simulink model "Ultrafiltration"  (R2025b)
settings: Solver=FixedStepAuto  StartTime=0.0  StopTime=1440  FixedStep=1  RelTol=1e-3
InitFcn:
  | initUF
  | tic;
StartFcn:
  | disp("Start...")
StopFcn:
  | disp("Stop...")
  | fprintf("SimTime: %.02f min", toc/60)
values from neighbouring files (symbols this model uses):
  BW_Max_Time = 90    [initUF.m]
  BW_Max_Vol_gal = 5000    [initUF.m]
  CEB_Max_Time = 1000    [initUF.m]
  CEB_Max_Vol_gal = 5000    [initUF.m]
  CIP_Max_Time = 15000    [initUF.m]
undefined symbols (not defined in the file or in its folder): LUT
libraries: simulink x30
(part 2 of 5)

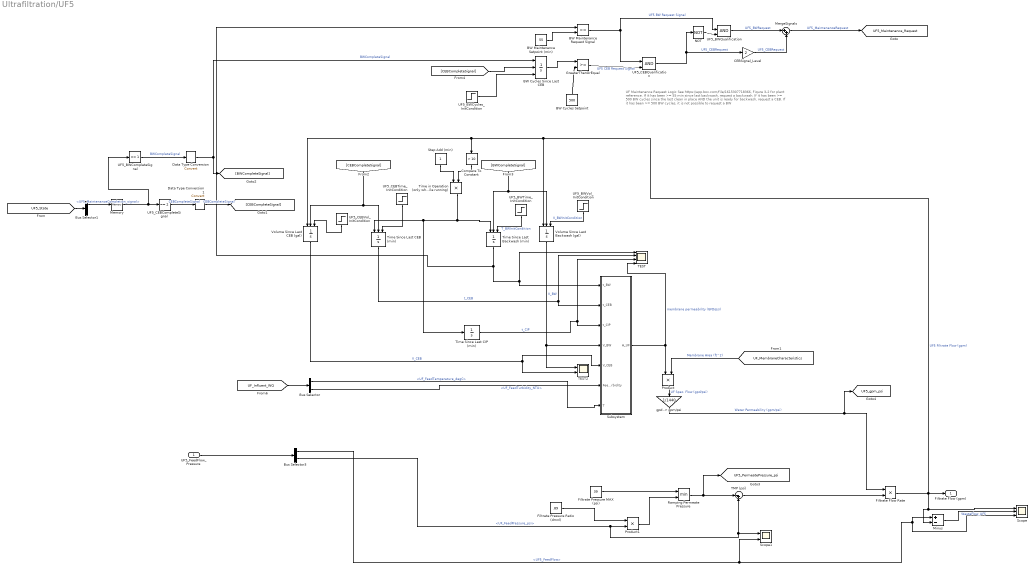
== system Ultrafiltration/UF5 ==
  note: UF Maintenance Request Logic
      | See https://app.box.com/file/1615307718366, Figure 3-2 for plant reference.
      |
      | If it has been >= 55 min since last backwash, request a backwash.
      | If it has been >= 500 BW cycles since the last clean in place AND the unit is ready for backwash, request a CEB.
      | If it has been >= 500 BW cycles, it is not possible to request a BW
  UF5_FeedFlow_Pressure : Inport
  BW Cycles Setpoint : Constant  Value=500
  BW Cycles Since Last CEB : Integrator  ExternalReset=rising  InitialConditionSource=external  InitialCondition=5
  BW Maintenance Request Signal : RelationalOperator  OutDataTypeStr=boolean  RndMeth=Simplest  InputSameDT=off
  BW Maintenance Setpoint (min) : Constant  Value=55
  Bus Selector : BusSelector  OutputSignals=UF_FeedTemperature_degC,UF_FeedTurbidity_NTU
  Bus Selector1 : BusSelector  OutputSignals=UF5_MaintenanceCompletion_signal,UF5_OperationsState_signal
  Bus Selector3 : BusSelector  OutputSignals=UF5_FeedFlow,UF_FeedPressure_psi
  CEBSignal_Level : Gain  Gain=2  OutDataTypeStr=double
  Compare To Constant : simulink/Logic and Bit Operations/Compare To Constant  relop=>  const=10  OutDataTypeStr=boolean
  Data Type Conversion : DataTypeConversion  SaturateOnIntegerOverflow=off  RndMeth=Floor
  Data Type Conversion1 : DataTypeConversion  SaturateOnIntegerOverflow=off  RndMeth=Floor
  Filtrate Flow Rate : Product
  Filtrate Pressure MAX (psi) : Constant  Value=39
  Filtrate Pressure Ratio (dmnl) : Constant  Value=.89
  GreaterThanOrEqual : RelationalOperator  OutDataTypeStr=boolean  RndMeth=Simplest  InputSameDT=off
  Memory : Memory
  MergeSignals : Sum  Inputs=|++
  Minus : Sum  Inputs=+-
  NOT : Logic  Operator=NOT  IconShape=distinctive  AllPortsSameDT=off  OutDataTypeStr=boolean
  Product : Product
  Product1 : Product
  Ramping Permeate Pressure : MinMax  Inputs=2
  Scope : Scope  NumInputPorts=3
      settings: ActiveDisplayYMinimum=-126.71796384165732  ActiveDisplayYMaximum=1140.4616745749161  DataLoggingVariableName=ScopeData10
  Scope1 : Scope  NumInputPorts=2
      settings: ActiveDisplayYMinimum=-129.2228584451866  ActiveDisplayYMaximum=1163.0057260066797  DataLoggingVariableName=ScopeData11
  Step Add (min) : Constant
  Subsystem : Subsystem
  TEST : Scope  NumInputPorts=4
      settings: ActiveDisplayYMinimum=13.625  ActiveDisplayYMaximum=27.375  DataLoggingVariableName=ScopeData3
  TEST2 : Scope  NumInputPorts=2
      settings: ActiveDisplayYMinimum=-311929.86683332996  ActiveDisplayYMaximum=2.8073688014999703E+6  DataLoggingVariableName=ScopeData4
  TMP (psi) : Sum  Inputs=|-+
  Time Since Last Backwash (min) : Integrator  ExternalReset=level hold  InitialConditionSource=external  InitialCondition=26
  Time Since Last CEB (min) : Integrator  ExternalReset=level hold  InitialConditionSource=external  InitialCondition=4833
  Time Since Last CIP (min) : Integrator  InitialCondition=round(CIP_Max_Time*rand())
  Time in Operation (only while running) : Product
  UF5_BWCompleteSignal : simulink/Logic and Bit Operations/Compare To Constant  relop===  const=1  OutDataTypeStr=uint8
  UF5_BWCycles_InitCondition : Step  Before=round(500 * rand())  After=0  SampleTime=0
  UF5_BWQualification : Logic  IconShape=distinctive  AllPortsSameDT=off  OutDataTypeStr=boolean
  UF5_BWTime_InitCondition : Step  Before=round(BW_Max_Time*rand())  After=0  SampleTime=0
  UF5_BWVol_InitCondition : Step  Before=round(BW_Max_Vol_gal*rand())  After=0  SampleTime=0
  UF5_CEBCompleteSignal : simulink/Logic and Bit Operations/Compare To Constant  relop===  const=2  OutDataTypeStr=uint8
  UF5_CEBQualification : Logic  IconShape=distinctive  AllPortsSameDT=off  OutDataTypeStr=boolean
  UF5_CEBTime_InitCondition : Step  Before=round(CEB_Max_Time*rand())  After=0  SampleTime=0
  UF5_CEBVol_InitCondition : Step  Before=round(CEB_Max_Vol_gal*rand())  After=0  SampleTime=0
  Volume Since Last Backwash (gal) : Integrator  ExternalReset=level hold  InitialConditionSource=external  InitialCondition=34330
  Volume Since Last CEB (gal) : Integrator  ExternalReset=rising  InitialConditionSource=external  InitialCondition=2777254
  "gpd -> gpm/psi" : Gain  Gain=1/1440
  Filtrate Flow (gpm) : Outport
  tag scope: UF5_Maintenance_Request=global, UF5_PermeatePressure_psi=global, UF5_gpm_psi=global
  wires:
  Volume Since Last Backwash (gal)/1 -> Subsystem/4(V_BW), TEST2/1  "V_BW"
  Time Since Last Backwash (min)/1 -> BW Maintenance Request Signal/1, Subsystem/1(t_BW), TEST/1
  Product/1 -> "gpd -> gpm/psi"/1  "UF Spec. Flow (gpd/psi)"
  [UF_MembraneCharacteristics] -> Product/2  "Membrane Area (ft^2)"
  "gpd -> gpm/psi"/1 -> Filtrate Flow Rate/1, [UF5_gpm_psi]  "Water Permeability (gpm/psi)"
  Time in Operation (only while running)/1 -> Time Since Last Backwash (min)/1, Time Since Last CEB (min)/1, Time Since Last CIP (min)/1
  Filtrate Flow Rate/1 -> Scope/1, Minus/2, Volume Since Last Backwash (gal)/1, Volume Since Last CEB (gal)/1, Compare To Constant/1, Filtrate Flow (gpm)/1  "UF5 Filtrate Flow (gpm)"
  Time Since Last CEB (min)/1 -> Subsystem/2(t_CEB), TEST/2  "t_CEB"
  Volume Since Last CEB (gal)/1 -> Subsystem/5(V_CEB), TEST2/2  "V_CEB"
  Time Since Last CIP (min)/1 -> Subsystem/3(t_CIP), TEST/3  "t_CIP"
  Filtrate Pressure MAX (psi)/1 -> Ramping Permeate Pressure/1
  [UF_Influent_WQ] -> Bus Selector/1
  Bus Selector/1 -> Subsystem/7(T)  "<UF_FeedTemperature_degC>"
  UF5_FeedFlow_Pressure/1 -> Bus Selector3/1
  Filtrate Pressure Ratio (dmnl)/1 -> Product1/1
  Product1/1 -> Ramping Permeate Pressure/2
  Ramping Permeate Pressure/1 -> [UF5_PermeatePressure_psi], TMP (psi)/1
  TMP (psi)/1 -> Filtrate Flow Rate/2
  BW Maintenance Setpoint (min)/1 -> BW Maintenance Request Signal/2
  BW Cycles Since Last CEB/1 -> GreaterThanOrEqual/1
  BW Cycles Setpoint/1 -> GreaterThanOrEqual/2
  Bus Selector/2 -> Subsystem/6(Feed Turbidity)  "<UF_FeedTurbidity_NTU>"
  [UF5_State] -> Bus Selector1/1
  MergeSignals/1 -> [UF5_Maintenance_Request]  "UF5_MaintenanceRequest"
  UF5_CEBCompleteSignal/1 -> Data Type Conversion1/1  "CEBCompleteSignal"
  [CEBCompleteSignal] -> Volume Since Last CEB (gal)/2, Time Since Last CEB (min)/2
  Data Type Conversion/1 -> [BWCompleteSignal], BW Cycles Since Last CEB/1  "BWCompleteSignal"
  [BWCompleteSignal] -> Volume Since Last Backwash (gal)/2, Time Since Last Backwash (min)/2
  [CEBCompleteSignal] -> BW Cycles Since Last CEB/2
  Bus Selector1/1 -> Memory/1  "<UF5_MaintenanceCompletion_signal>"
  UF5_BWCompleteSignal/1 -> Data Type Conversion/1  "BWCompleteSignal"
  Data Type Conversion1/1 -> [CEBCompleteSignal]  "CEBCompleteSignal"
  UF5_BWCycles_InitCondition/1 -> BW Cycles Since Last CEB/3
  Subsystem/1(A_UF) -> TEST/4, Product/1  "membrane permeability (GFD/psi)"
  UF5_BWTime_InitCondition/1 -> Time Since Last Backwash (min)/3  "T_BWInitCondition"
  UF5_CEBVol_InitCondition/1 -> Volume Since Last CEB (gal)/3
  UF5_CEBTime_InitCondition/1 -> Time Since Last CEB (min)/3
  UF5_BWVol_InitCondition/1 -> Volume Since Last Backwash (gal)/3  "V_BWInitCondition"
  Step Add (min)/1 -> Time in Operation (only while running)/1
  Compare To Constant/1 -> Time in Operation (only while running)/2
  Memory/1 -> UF5_BWCompleteSignal/1, UF5_CEBCompleteSignal/1
  UF5_BWQualification/1 -> MergeSignals/1  "UF5_BWRequest"
  GreaterThanOrEqual/1 -> UF5_CEBQualification/2  "UF5 CEB Request Signal"
  UF5_CEBQualification/1 -> CEBSignal_Level/1, NOT/1  "UF5_CEBRequest"
  BW Maintenance Request Signal/1 -> UF5_BWQualification/1, UF5_CEBQualification/1  "UF5 BW Request Signal"
  NOT/1 -> UF5_BWQualification/2
  CEBSignal_Level/1 -> MergeSignals/2  "UF5_CEBRequest"
  Bus Selector3/1 -> Scope1/2, Minus/1, Scope/3  "<UF5_FeedFlow>"
  Bus Selector3/2 -> TMP (psi)/2, Scope1/1, Product1/2  "<UF_FeedPressure_psi>"
  Minus/1 -> Scope/2  "WasteFlow_UF5"

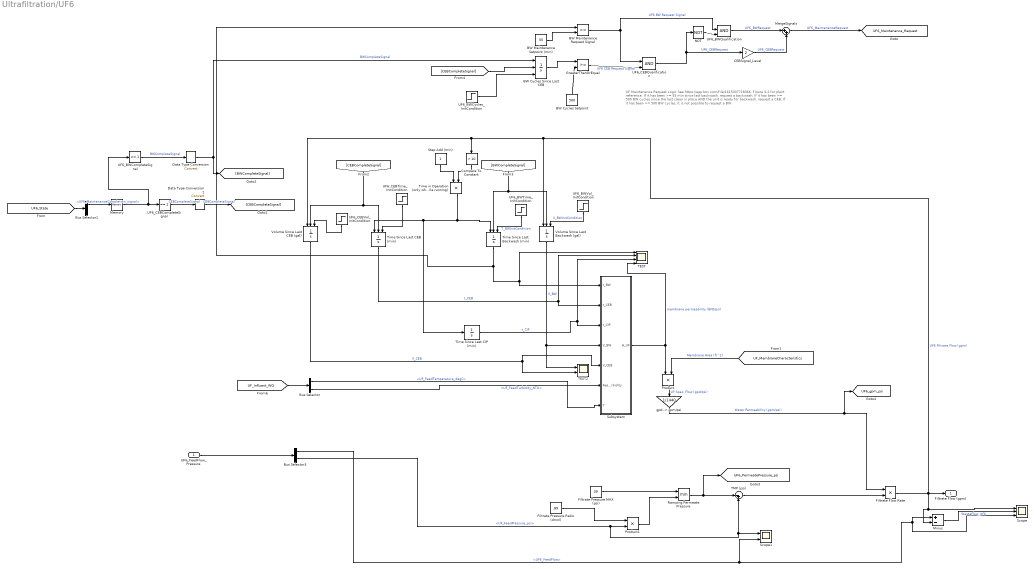
== system Ultrafiltration/UF6 ==
  note: UF Maintenance Request Logic
      | See https://app.box.com/file/1615307718366, Figure 3-2 for plant reference.
      |
      | If it has been >= 55 min since last backwash, request a backwash.
      | If it has been >= 500 BW cycles since the last clean in place AND the unit is ready for backwash, request a CEB.
      | If it has been >= 500 BW cycles, it is not possible to request a BW
  UF6_FeedFlow_Pressure : Inport
  BW Cycles Setpoint : Constant  Value=500
  BW Cycles Since Last CEB : Integrator  ExternalReset=rising  InitialConditionSource=external  InitialCondition=5
  BW Maintenance Request Signal : RelationalOperator  OutDataTypeStr=boolean  RndMeth=Simplest  InputSameDT=off
  BW Maintenance Setpoint (min) : Constant  Value=55
  Bus Selector : BusSelector  OutputSignals=UF_FeedTemperature_degC,UF_FeedTurbidity_NTU
  Bus Selector1 : BusSelector  OutputSignals=UF6_MaintenanceCompletion_signal,UF6_OperationsState_signal
  Bus Selector3 : BusSelector  OutputSignals=UF6_FeedFlow,UF_FeedPressure_psi
  CEBSignal_Level : Gain  Gain=2  OutDataTypeStr=double
  Compare To Constant : simulink/Logic and Bit Operations/Compare To Constant  relop=>  const=10  OutDataTypeStr=boolean
  Data Type Conversion : DataTypeConversion  SaturateOnIntegerOverflow=off  RndMeth=Floor
  Data Type Conversion1 : DataTypeConversion  SaturateOnIntegerOverflow=off  RndMeth=Floor
  Filtrate Flow Rate : Product
  Filtrate Pressure MAX (psi) : Constant  Value=39
  Filtrate Pressure Ratio (dmnl) : Constant  Value=.89
  GreaterThanOrEqual : RelationalOperator  OutDataTypeStr=boolean  RndMeth=Simplest  InputSameDT=off
  Memory : Memory
  MergeSignals : Sum  Inputs=|++
  Minus : Sum  Inputs=+-
  NOT : Logic  Operator=NOT  IconShape=distinctive  AllPortsSameDT=off  OutDataTypeStr=boolean
  Product : Product
  Product1 : Product
  Ramping Permeate Pressure : MinMax  Inputs=2
  Scope : Scope  NumInputPorts=3
      settings: ActiveDisplayYMinimum=-126.71796384165732  ActiveDisplayYMaximum=1140.4616745749161  DataLoggingVariableName=ScopeData10
  Scope1 : Scope  NumInputPorts=2
      settings: ActiveDisplayYMinimum=-129.2228584451866  ActiveDisplayYMaximum=1163.0057260066797  DataLoggingVariableName=ScopeData11
  Step Add (min) : Constant
  Subsystem : Subsystem
  TEST : Scope  NumInputPorts=4
      settings: ActiveDisplayYMinimum=13.625  ActiveDisplayYMaximum=27.375  DataLoggingVariableName=ScopeData3
  TEST2 : Scope  NumInputPorts=2
      settings: ActiveDisplayYMinimum=-311929.86683332996  ActiveDisplayYMaximum=2.8073688014999703E+6  DataLoggingVariableName=ScopeData4
  TMP (psi) : Sum  Inputs=|-+
  Time Since Last Backwash (min) : Integrator  ExternalReset=level hold  InitialConditionSource=external  InitialCondition=26
  Time Since Last CEB (min) : Integrator  ExternalReset=level hold  InitialConditionSource=external  InitialCondition=4833
  Time Since Last CIP (min) : Integrator  InitialCondition=round(CIP_Max_Time*rand())
  Time in Operation (only while running) : Product
  UF6_BWCompleteSignal : simulink/Logic and Bit Operations/Compare To Constant  relop===  const=1  OutDataTypeStr=uint8
  UF6_BWCycles_InitCondition : Step  Before=round(500 * rand())  After=0  SampleTime=0
  UF6_BWQualification : Logic  IconShape=distinctive  AllPortsSameDT=off  OutDataTypeStr=boolean
  UF6_BWTime_InitCondition : Step  Before=round(BW_Max_Time*rand())  After=0  SampleTime=0
  UF6_BWVol_InitCondition : Step  Before=round(BW_Max_Vol_gal*rand())  After=0  SampleTime=0
  UF6_CEBCompleteSignal : simulink/Logic and Bit Operations/Compare To Constant  relop===  const=2  OutDataTypeStr=uint8
  UF6_CEBQualification : Logic  IconShape=distinctive  AllPortsSameDT=off  OutDataTypeStr=boolean
  UF6_CEBTime_InitCondition : Step  Before=round(CEB_Max_Time*rand())  After=0  SampleTime=0
  UF6_CEBVol_InitCondition : Step  Before=round(CEB_Max_Vol_gal*rand())  After=0  SampleTime=0
  Volume Since Last Backwash (gal) : Integrator  ExternalReset=level hold  InitialConditionSource=external  InitialCondition=34330
  Volume Since Last CEB (gal) : Integrator  ExternalReset=rising  InitialConditionSource=external  InitialCondition=2777254
  "gpd -> gpm/psi" : Gain  Gain=1/1440
  Filtrate Flow (gpm) : Outport
  tag scope: UF6_Maintenance_Request=global, UF6_PermeatePressure_psi=global, UF6_gpm_psi=global
  wires:
  Volume Since Last Backwash (gal)/1 -> Subsystem/4(V_BW), TEST2/1  "V_BW"
  Time Since Last Backwash (min)/1 -> BW Maintenance Request Signal/1, Subsystem/1(t_BW), TEST/1
  Product/1 -> "gpd -> gpm/psi"/1  "UF Spec. Flow (gpd/psi)"
  [UF_MembraneCharacteristics] -> Product/2  "Membrane Area (ft^2)"
  "gpd -> gpm/psi"/1 -> Filtrate Flow Rate/1, [UF6_gpm_psi]  "Water Permeability (gpm/psi)"
  Time in Operation (only while running)/1 -> Time Since Last Backwash (min)/1, Time Since Last CEB (min)/1, Time Since Last CIP (min)/1
  Filtrate Flow Rate/1 -> Scope/1, Minus/2, Volume Since Last Backwash (gal)/1, Volume Since Last CEB (gal)/1, Compare To Constant/1, Filtrate Flow (gpm)/1  "UF6 Filtrate Flow (gpm)"
  Time Since Last CEB (min)/1 -> Subsystem/2(t_CEB), TEST/2  "t_CEB"
  Volume Since Last CEB (gal)/1 -> Subsystem/5(V_CEB), TEST2/2  "V_CEB"
  Time Since Last CIP (min)/1 -> Subsystem/3(t_CIP), TEST/3  "t_CIP"
  Filtrate Pressure MAX (psi)/1 -> Ramping Permeate Pressure/1
  [UF_Influent_WQ] -> Bus Selector/1
  Bus Selector/1 -> Subsystem/7(T)  "<UF_FeedTemperature_degC>"
  UF6_FeedFlow_Pressure/1 -> Bus Selector3/1
  Filtrate Pressure Ratio (dmnl)/1 -> Product1/1
  Product1/1 -> Ramping Permeate Pressure/2
  Ramping Permeate Pressure/1 -> [UF6_PermeatePressure_psi], TMP (psi)/1
  TMP (psi)/1 -> Filtrate Flow Rate/2
  BW Maintenance Setpoint (min)/1 -> BW Maintenance Request Signal/2
  BW Cycles Since Last CEB/1 -> GreaterThanOrEqual/1
  BW Cycles Setpoint/1 -> GreaterThanOrEqual/2
  Bus Selector/2 -> Subsystem/6(Feed Turbidity)  "<UF_FeedTurbidity_NTU>"
  [UF6_State] -> Bus Selector1/1
  MergeSignals/1 -> [UF6_Maintenance_Request]  "UF6_MaintenanceRequest"
  UF6_CEBCompleteSignal/1 -> Data Type Conversion1/1  "CEBCompleteSignal"
  [CEBCompleteSignal] -> Volume Since Last CEB (gal)/2, Time Since Last CEB (min)/2
  Data Type Conversion/1 -> [BWCompleteSignal], BW Cycles Since Last CEB/1  "BWCompleteSignal"
  [BWCompleteSignal] -> Volume Since Last Backwash (gal)/2, Time Since Last Backwash (min)/2
  [CEBCompleteSignal] -> BW Cycles Since Last CEB/2
  Bus Selector1/1 -> Memory/1  "<UF6_MaintenanceCompletion_signal>"
  UF6_BWCompleteSignal/1 -> Data Type Conversion/1  "BWCompleteSignal"
  Data Type Conversion1/1 -> [CEBCompleteSignal]  "CEBCompleteSignal"
  UF6_BWCycles_InitCondition/1 -> BW Cycles Since Last CEB/3
  Subsystem/1(A_UF) -> TEST/4, Product/1  "membrane permeability (GFD/psi)"
  UF6_BWTime_InitCondition/1 -> Time Since Last Backwash (min)/3  "T_BWInitCondition"
  UF6_CEBVol_InitCondition/1 -> Volume Since Last CEB (gal)/3
  UF6_CEBTime_InitCondition/1 -> Time Since Last CEB (min)/3
  UF6_BWVol_InitCondition/1 -> Volume Since Last Backwash (gal)/3  "V_BWInitCondition"
  Step Add (min)/1 -> Time in Operation (only while running)/1
  Compare To Constant/1 -> Time in Operation (only while running)/2
  Memory/1 -> UF6_BWCompleteSignal/1, UF6_CEBCompleteSignal/1
  UF6_BWQualification/1 -> MergeSignals/1  "UF6_BWRequest"
  GreaterThanOrEqual/1 -> UF6_CEBQualification/2  "UF6 CEB Request Signal"
  UF6_CEBQualification/1 -> CEBSignal_Level/1, NOT/1  "UF6_CEBRequest"
  BW Maintenance Request Signal/1 -> UF6_BWQualification/1, UF6_CEBQualification/1  "UF6 BW Request Signal"
  NOT/1 -> UF6_BWQualification/2
  CEBSignal_Level/1 -> MergeSignals/2  "UF6_CEBRequest"
  Bus Selector3/1 -> Scope1/2, Minus/1, Scope/3  "<UF6_FeedFlow>"
  Bus Selector3/2 -> TMP (psi)/2, Scope1/1, Product1/2  "<UF_FeedPressure_psi>"
  Minus/1 -> Scope/2  "WasteFlow_UF6"

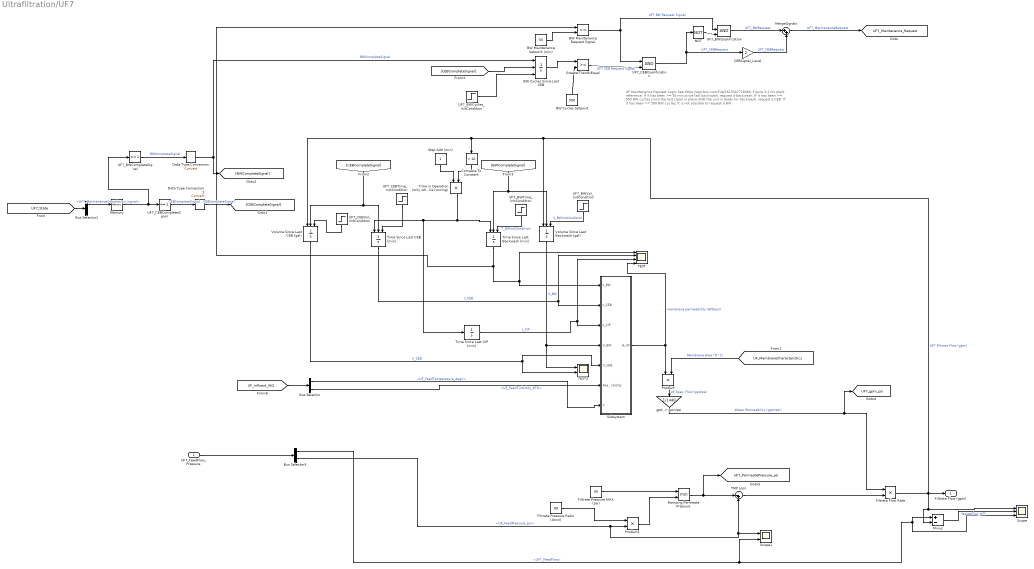
== system Ultrafiltration/UF7 ==
  note: UF Maintenance Request Logic
      | See https://app.box.com/file/1615307718366, Figure 3-2 for plant reference.
      |
      | If it has been >= 55 min since last backwash, request a backwash.
      | If it has been >= 500 BW cycles since the last clean in place AND the unit is ready for backwash, request a CEB.
      | If it has been >= 500 BW cycles, it is not possible to request a BW
  UF7_FeedFlow_Pressure : Inport
  BW Cycles Setpoint : Constant  Value=500
  BW Cycles Since Last CEB : Integrator  ExternalReset=rising  InitialConditionSource=external  InitialCondition=5
  BW Maintenance Request Signal : RelationalOperator  OutDataTypeStr=boolean  RndMeth=Simplest  InputSameDT=off
  BW Maintenance Setpoint (min) : Constant  Value=55
  Bus Selector : BusSelector  OutputSignals=UF_FeedTemperature_degC,UF_FeedTurbidity_NTU
  Bus Selector1 : BusSelector  OutputSignals=UF7_MaintenanceCompletion_signal,UF7_OperationsState_signal
  Bus Selector3 : BusSelector  OutputSignals=UF7_FeedFlow,UF_FeedPressure_psi
  CEBSignal_Level : Gain  Gain=2  OutDataTypeStr=double
  Compare To Constant : simulink/Logic and Bit Operations/Compare To Constant  relop=>  const=10  OutDataTypeStr=boolean
  Data Type Conversion : DataTypeConversion  SaturateOnIntegerOverflow=off  RndMeth=Floor
  Data Type Conversion1 : DataTypeConversion  SaturateOnIntegerOverflow=off  RndMeth=Floor
  Filtrate Flow Rate : Product
  Filtrate Pressure MAX (psi) : Constant  Value=39
  Filtrate Pressure Ratio (dmnl) : Constant  Value=.89
  GreaterThanOrEqual : RelationalOperator  OutDataTypeStr=boolean  RndMeth=Simplest  InputSameDT=off
  Memory : Memory
  MergeSignals : Sum  Inputs=|++
  Minus : Sum  Inputs=+-
  NOT : Logic  Operator=NOT  IconShape=distinctive  AllPortsSameDT=off  OutDataTypeStr=boolean
  Product : Product
  Product1 : Product
  Ramping Permeate Pressure : MinMax  Inputs=2
  Scope : Scope  NumInputPorts=3
      settings: ActiveDisplayYMinimum=-126.71796384165732  ActiveDisplayYMaximum=1140.4616745749161  DataLoggingVariableName=ScopeData10
  Scope1 : Scope  NumInputPorts=2
      settings: ActiveDisplayYMinimum=-129.2228584451866  ActiveDisplayYMaximum=1163.0057260066797  DataLoggingVariableName=ScopeData11
  Step Add (min) : Constant
  Subsystem : Subsystem
  TEST : Scope  NumInputPorts=4
      settings: ActiveDisplayYMinimum=13.625  ActiveDisplayYMaximum=27.375  DataLoggingVariableName=ScopeData3
  TEST2 : Scope  NumInputPorts=2
      settings: ActiveDisplayYMinimum=-311929.86683332996  ActiveDisplayYMaximum=2.8073688014999703E+6  DataLoggingVariableName=ScopeData4
  TMP (psi) : Sum  Inputs=|-+
  Time Since Last Backwash (min) : Integrator  ExternalReset=level hold  InitialConditionSource=external  InitialCondition=26
  Time Since Last CEB (min) : Integrator  ExternalReset=level hold  InitialConditionSource=external  InitialCondition=4833
  Time Since Last CIP (min) : Integrator  InitialCondition=round(CIP_Max_Time*rand())
  Time in Operation (only while running) : Product
  UF7_BWCompleteSignal : simulink/Logic and Bit Operations/Compare To Constant  relop===  const=1  OutDataTypeStr=uint8
  UF7_BWCycles_InitCondition : Step  Before=round(500 * rand())  After=0  SampleTime=0
  UF7_BWQualification : Logic  IconShape=distinctive  AllPortsSameDT=off  OutDataTypeStr=boolean
  UF7_BWTime_InitCondition : Step  Before=round(BW_Max_Time*rand())  After=0  SampleTime=0
  UF7_BWVol_InitCondition : Step  Before=round(BW_Max_Vol_gal*rand())  After=0  SampleTime=0
  UF7_CEBCompleteSignal : simulink/Logic and Bit Operations/Compare To Constant  relop===  const=2  OutDataTypeStr=uint8
  UF7_CEBQualification : Logic  IconShape=distinctive  AllPortsSameDT=off  OutDataTypeStr=boolean
  UF7_CEBTime_InitCondition : Step  Before=round(CEB_Max_Time*rand())  After=0  SampleTime=0
  UF7_CEBVol_InitCondition : Step  Before=round(CEB_Max_Vol_gal*rand())  After=0  SampleTime=0
  Volume Since Last Backwash (gal) : Integrator  ExternalReset=level hold  InitialConditionSource=external  InitialCondition=34330
  Volume Since Last CEB (gal) : Integrator  ExternalReset=rising  InitialConditionSource=external  InitialCondition=2777254
  "gpd -> gpm/psi" : Gain  Gain=1/1440
  Filtrate Flow (gpm) : Outport
  tag scope: UF7_Maintenance_Request=global, UF7_PermeatePressure_psi=global, UF7_gpm_psi=global
  wires:
  Volume Since Last Backwash (gal)/1 -> Subsystem/4(V_BW), TEST2/1  "V_BW"
  Time Since Last Backwash (min)/1 -> BW Maintenance Request Signal/1, Subsystem/1(t_BW), TEST/1
  Product/1 -> "gpd -> gpm/psi"/1  "UF Spec. Flow (gpd/psi)"
  [UF_MembraneCharacteristics] -> Product/2  "Membrane Area (ft^2)"
  "gpd -> gpm/psi"/1 -> Filtrate Flow Rate/1, [UF7_gpm_psi]  "Water Permeability (gpm/psi)"
  Time in Operation (only while running)/1 -> Time Since Last Backwash (min)/1, Time Since Last CEB (min)/1, Time Since Last CIP (min)/1
  Filtrate Flow Rate/1 -> Scope/1, Minus/2, Volume Since Last Backwash (gal)/1, Volume Since Last CEB (gal)/1, Compare To Constant/1, Filtrate Flow (gpm)/1  "UF7 Filtrate Flow (gpm)"
  Time Since Last CEB (min)/1 -> Subsystem/2(t_CEB), TEST/2  "t_CEB"
  Volume Since Last CEB (gal)/1 -> Subsystem/5(V_CEB), TEST2/2  "V_CEB"
  Time Since Last CIP (min)/1 -> Subsystem/3(t_CIP), TEST/3  "t_CIP"
  Filtrate Pressure MAX (psi)/1 -> Ramping Permeate Pressure/1
  [UF_Influent_WQ] -> Bus Selector/1
  Bus Selector/1 -> Subsystem/7(T)  "<UF_FeedTemperature_degC>"
  UF7_FeedFlow_Pressure/1 -> Bus Selector3/1
  Filtrate Pressure Ratio (dmnl)/1 -> Product1/1
  Product1/1 -> Ramping Permeate Pressure/2
  Ramping Permeate Pressure/1 -> [UF7_PermeatePressure_psi], TMP (psi)/1
  TMP (psi)/1 -> Filtrate Flow Rate/2
  BW Maintenance Setpoint (min)/1 -> BW Maintenance Request Signal/2
  BW Cycles Since Last CEB/1 -> GreaterThanOrEqual/1
  BW Cycles Setpoint/1 -> GreaterThanOrEqual/2
  Bus Selector/2 -> Subsystem/6(Feed Turbidity)  "<UF_FeedTurbidity_NTU>"
  [UF7_State] -> Bus Selector1/1
  MergeSignals/1 -> [UF7_Maintenance_Request]  "UF7_MaintenanceRequest"
  UF7_CEBCompleteSignal/1 -> Data Type Conversion1/1  "CEBCompleteSignal"
  [CEBCompleteSignal] -> Volume Since Last CEB (gal)/2, Time Since Last CEB (min)/2
  Data Type Conversion/1 -> [BWCompleteSignal], BW Cycles Since Last CEB/1  "BWCompleteSignal"
  [BWCompleteSignal] -> Volume Since Last Backwash (gal)/2, Time Since Last Backwash (min)/2
  [CEBCompleteSignal] -> BW Cycles Since Last CEB/2
  Bus Selector1/1 -> Memory/1  "<UF7_MaintenanceCompletion_signal>"
  UF7_BWCompleteSignal/1 -> Data Type Conversion/1  "BWCompleteSignal"
  Data Type Conversion1/1 -> [CEBCompleteSignal]  "CEBCompleteSignal"
  UF7_BWCycles_InitCondition/1 -> BW Cycles Since Last CEB/3
  Subsystem/1(A_UF) -> TEST/4, Product/1  "membrane permeability (GFD/psi)"
  UF7_BWTime_InitCondition/1 -> Time Since Last Backwash (min)/3  "T_BWInitCondition"
  UF7_CEBVol_InitCondition/1 -> Volume Since Last CEB (gal)/3
  UF7_CEBTime_InitCondition/1 -> Time Since Last CEB (min)/3
  UF7_BWVol_InitCondition/1 -> Volume Since Last Backwash (gal)/3  "V_BWInitCondition"
  Step Add (min)/1 -> Time in Operation (only while running)/1
  Compare To Constant/1 -> Time in Operation (only while running)/2
  Memory/1 -> UF7_BWCompleteSignal/1, UF7_CEBCompleteSignal/1
  UF7_BWQualification/1 -> MergeSignals/1  "UF7_BWRequest"
  GreaterThanOrEqual/1 -> UF7_CEBQualification/2  "UF7 CEB Request Signal"
  UF7_CEBQualification/1 -> CEBSignal_Level/1, NOT/1  "UF7_CEBRequest"
  BW Maintenance Request Signal/1 -> UF7_BWQualification/1, UF7_CEBQualification/1  "UF7 BW Request Signal"
  NOT/1 -> UF7_BWQualification/2
  CEBSignal_Level/1 -> MergeSignals/2  "UF7_CEBRequest"
  Bus Selector3/1 -> Scope1/2, Minus/1, Scope/3  "<UF7_FeedFlow>"
  Bus Selector3/2 -> TMP (psi)/2, Scope1/1, Product1/2  "<UF_FeedPressure_psi>"
  Minus/1 -> Scope/2  "WasteFlow_UF7"

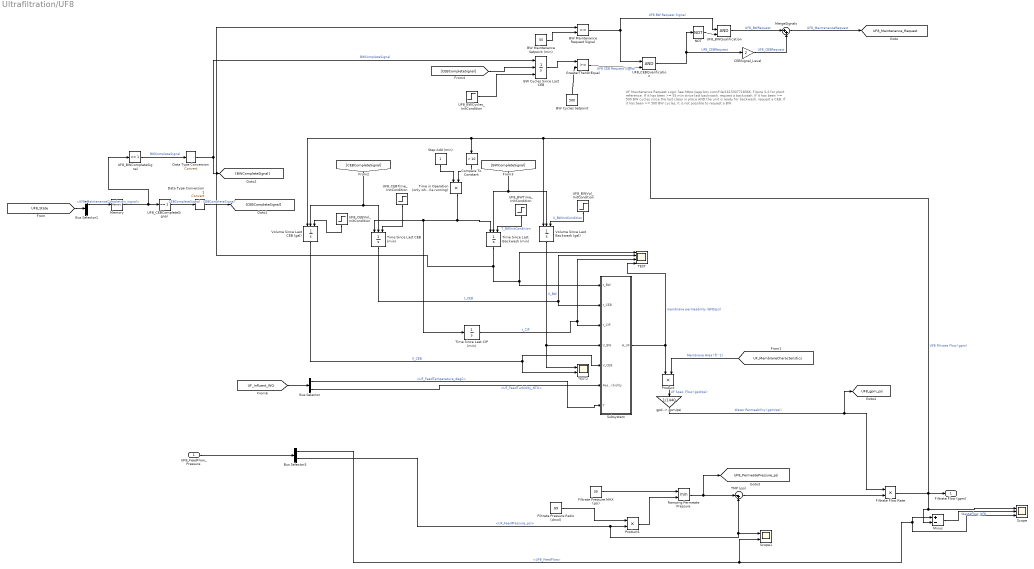
== system Ultrafiltration/UF8 ==
  note: UF Maintenance Request Logic
      | See https://app.box.com/file/1615307718366, Figure 3-2 for plant reference.
      |
      | If it has been >= 55 min since last backwash, request a backwash.
      | If it has been >= 500 BW cycles since the last clean in place AND the unit is ready for backwash, request a CEB.
      | If it has been >= 500 BW cycles, it is not possible to request a BW
  UF8_FeedFlow_Pressure : Inport
  BW Cycles Setpoint : Constant  Value=500
  BW Cycles Since Last CEB : Integrator  ExternalReset=rising  InitialConditionSource=external  InitialCondition=5
  BW Maintenance Request Signal : RelationalOperator  OutDataTypeStr=boolean  RndMeth=Simplest  InputSameDT=off
  BW Maintenance Setpoint (min) : Constant  Value=55
  Bus Selector : BusSelector  OutputSignals=UF_FeedTemperature_degC,UF_FeedTurbidity_NTU
  Bus Selector1 : BusSelector  OutputSignals=UF8_MaintenanceCompletion_signal,UF8_OperationsState_signal
  Bus Selector3 : BusSelector  OutputSignals=UF8_FeedFlow,UF_FeedPressure_psi
  CEBSignal_Level : Gain  Gain=2  OutDataTypeStr=double
  Compare To Constant : simulink/Logic and Bit Operations/Compare To Constant  relop=>  const=10  OutDataTypeStr=boolean
  Data Type Conversion : DataTypeConversion  SaturateOnIntegerOverflow=off  RndMeth=Floor
  Data Type Conversion1 : DataTypeConversion  SaturateOnIntegerOverflow=off  RndMeth=Floor
  Filtrate Flow Rate : Product
  Filtrate Pressure MAX (psi) : Constant  Value=39
  Filtrate Pressure Ratio (dmnl) : Constant  Value=.89
  GreaterThanOrEqual : RelationalOperator  OutDataTypeStr=boolean  RndMeth=Simplest  InputSameDT=off
  Memory : Memory
  MergeSignals : Sum  Inputs=|++
  Minus : Sum  Inputs=+-
  NOT : Logic  Operator=NOT  IconShape=distinctive  AllPortsSameDT=off  OutDataTypeStr=boolean
  Product : Product
  Product1 : Product
  Ramping Permeate Pressure : MinMax  Inputs=2
  Scope : Scope  NumInputPorts=3
      settings: ActiveDisplayYMinimum=-126.71796384165732  ActiveDisplayYMaximum=1140.4616745749161  DataLoggingVariableName=ScopeData10
  Scope1 : Scope  NumInputPorts=2
      settings: ActiveDisplayYMinimum=-129.2228584451866  ActiveDisplayYMaximum=1163.0057260066797  DataLoggingVariableName=ScopeData11
  Step Add (min) : Constant
  Subsystem : Subsystem
  TEST : Scope  NumInputPorts=4
      settings: ActiveDisplayYMinimum=13.625  ActiveDisplayYMaximum=27.375  DataLoggingVariableName=ScopeData3
  TEST2 : Scope  NumInputPorts=2
      settings: ActiveDisplayYMinimum=-311929.86683332996  ActiveDisplayYMaximum=2.8073688014999703E+6  DataLoggingVariableName=ScopeData4
  TMP (psi) : Sum  Inputs=|-+
  Time Since Last Backwash (min) : Integrator  ExternalReset=level hold  InitialConditionSource=external  InitialCondition=26
  Time Since Last CEB (min) : Integrator  ExternalReset=level hold  InitialConditionSource=external  InitialCondition=4833
  Time Since Last CIP (min) : Integrator  InitialCondition=round(CIP_Max_Time*rand())
  Time in Operation (only while running) : Product
  UF8_BWCompleteSignal : simulink/Logic and Bit Operations/Compare To Constant  relop===  const=1  OutDataTypeStr=uint8
  UF8_BWCycles_InitCondition : Step  Before=round(500 * rand())  After=0  SampleTime=0
  UF8_BWQualification : Logic  IconShape=distinctive  AllPortsSameDT=off  OutDataTypeStr=boolean
  UF8_BWTime_InitCondition : Step  Before=round(BW_Max_Time*rand())  After=0  SampleTime=0
  UF8_BWVol_InitCondition : Step  Before=round(BW_Max_Vol_gal*rand())  After=0  SampleTime=0
  UF8_CEBCompleteSignal : simulink/Logic and Bit Operations/Compare To Constant  relop===  const=2  OutDataTypeStr=uint8
  UF8_CEBQualification : Logic  IconShape=distinctive  AllPortsSameDT=off  OutDataTypeStr=boolean
  UF8_CEBTime_InitCondition : Step  Before=round(CEB_Max_Time*rand())  After=0  SampleTime=0
  UF8_CEBVol_InitCondition : Step  Before=round(CEB_Max_Vol_gal*rand())  After=0  SampleTime=0
  Volume Since Last Backwash (gal) : Integrator  ExternalReset=level hold  InitialConditionSource=external  InitialCondition=34330
  Volume Since Last CEB (gal) : Integrator  ExternalReset=rising  InitialConditionSource=external  InitialCondition=2777254
  "gpd -> gpm/psi" : Gain  Gain=1/1440
  Filtrate Flow (gpm) : Outport
  tag scope: UF8_Maintenance_Request=global, UF8_PermeatePressure_psi=global, UF8_gpm_psi=global
  wires:
  Volume Since Last Backwash (gal)/1 -> Subsystem/4(V_BW), TEST2/1  "V_BW"
  Time Since Last Backwash (min)/1 -> BW Maintenance Request Signal/1, Subsystem/1(t_BW), TEST/1
  Product/1 -> "gpd -> gpm/psi"/1  "UF Spec. Flow (gpd/psi)"
  [UF_MembraneCharacteristics] -> Product/2  "Membrane Area (ft^2)"
  "gpd -> gpm/psi"/1 -> Filtrate Flow Rate/1, [UF8_gpm_psi]  "Water Permeability (gpm/psi)"
  Time in Operation (only while running)/1 -> Time Since Last Backwash (min)/1, Time Since Last CEB (min)/1, Time Since Last CIP (min)/1
  Filtrate Flow Rate/1 -> Scope/1, Minus/2, Volume Since Last Backwash (gal)/1, Volume Since Last CEB (gal)/1, Compare To Constant/1, Filtrate Flow (gpm)/1  "UF8 Filtrate Flow (gpm)"
  Time Since Last CEB (min)/1 -> Subsystem/2(t_CEB), TEST/2  "t_CEB"
  Volume Since Last CEB (gal)/1 -> Subsystem/5(V_CEB), TEST2/2  "V_CEB"
  Time Since Last CIP (min)/1 -> Subsystem/3(t_CIP), TEST/3  "t_CIP"
  Filtrate Pressure MAX (psi)/1 -> Ramping Permeate Pressure/1
  [UF_Influent_WQ] -> Bus Selector/1
  Bus Selector/1 -> Subsystem/7(T)  "<UF_FeedTemperature_degC>"
  UF8_FeedFlow_Pressure/1 -> Bus Selector3/1
  Filtrate Pressure Ratio (dmnl)/1 -> Product1/1
  Product1/1 -> Ramping Permeate Pressure/2
  Ramping Permeate Pressure/1 -> [UF8_PermeatePressure_psi], TMP (psi)/1
  TMP (psi)/1 -> Filtrate Flow Rate/2
  BW Maintenance Setpoint (min)/1 -> BW Maintenance Request Signal/2
  BW Cycles Since Last CEB/1 -> GreaterThanOrEqual/1
  BW Cycles Setpoint/1 -> GreaterThanOrEqual/2
  Bus Selector/2 -> Subsystem/6(Feed Turbidity)  "<UF_FeedTurbidity_NTU>"
  [UF8_State] -> Bus Selector1/1
  MergeSignals/1 -> [UF8_Maintenance_Request]  "UF8_MaintenanceRequest"
  UF8_CEBCompleteSignal/1 -> Data Type Conversion1/1  "CEBCompleteSignal"
  [CEBCompleteSignal] -> Volume Since Last CEB (gal)/2, Time Since Last CEB (min)/2
  Data Type Conversion/1 -> [BWCompleteSignal], BW Cycles Since Last CEB/1  "BWCompleteSignal"
  [BWCompleteSignal] -> Volume Since Last Backwash (gal)/2, Time Since Last Backwash (min)/2
  [CEBCompleteSignal] -> BW Cycles Since Last CEB/2
  Bus Selector1/1 -> Memory/1  "<UF8_MaintenanceCompletion_signal>"
  UF8_BWCompleteSignal/1 -> Data Type Conversion/1  "BWCompleteSignal"
  Data Type Conversion1/1 -> [CEBCompleteSignal]  "CEBCompleteSignal"
  UF8_BWCycles_InitCondition/1 -> BW Cycles Since Last CEB/3
  Subsystem/1(A_UF) -> TEST/4, Product/1  "membrane permeability (GFD/psi)"
  UF8_BWTime_InitCondition/1 -> Time Since Last Backwash (min)/3  "T_BWInitCondition"
  UF8_CEBVol_InitCondition/1 -> Volume Since Last CEB (gal)/3
  UF8_CEBTime_InitCondition/1 -> Time Since Last CEB (min)/3
  UF8_BWVol_InitCondition/1 -> Volume Since Last Backwash (gal)/3  "V_BWInitCondition"
  Step Add (min)/1 -> Time in Operation (only while running)/1
  Compare To Constant/1 -> Time in Operation (only while running)/2
  Memory/1 -> UF8_BWCompleteSignal/1, UF8_CEBCompleteSignal/1
  UF8_BWQualification/1 -> MergeSignals/1  "UF8_BWRequest"
  GreaterThanOrEqual/1 -> UF8_CEBQualification/2  "UF8 CEB Request Signal"
  UF8_CEBQualification/1 -> CEBSignal_Level/1, NOT/1  "UF8_CEBRequest"
  BW Maintenance Request Signal/1 -> UF8_BWQualification/1, UF8_CEBQualification/1  "UF8 BW Request Signal"
  NOT/1 -> UF8_BWQualification/2
  CEBSignal_Level/1 -> MergeSignals/2  "UF8_CEBRequest"
  Bus Selector3/1 -> Scope1/2, Minus/1, Scope/3  "<UF8_FeedFlow>"
  Bus Selector3/2 -> TMP (psi)/2, Scope1/1, Product1/2  "<UF_FeedPressure_psi>"
  Minus/1 -> Scope/2  "WasteFlow_UF8"

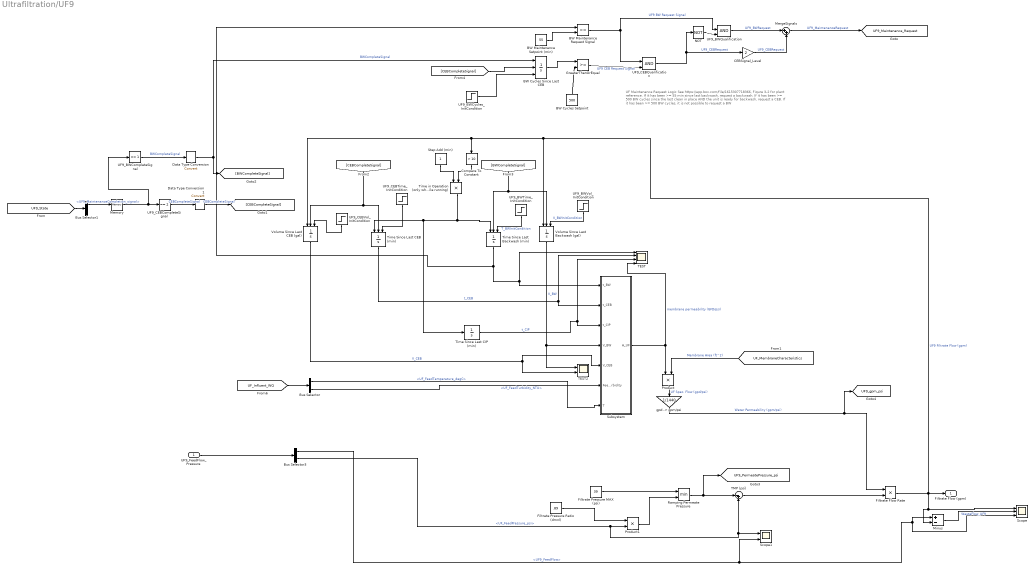
== system Ultrafiltration/UF9 ==
  note: UF Maintenance Request Logic
      | See https://app.box.com/file/1615307718366, Figure 3-2 for plant reference.
      |
      | If it has been >= 55 min since last backwash, request a backwash.
      | If it has been >= 500 BW cycles since the last clean in place AND the unit is ready for backwash, request a CEB.
      | If it has been >= 500 BW cycles, it is not possible to request a BW
  UF9_FeedFlow_Pressure : Inport
  BW Cycles Setpoint : Constant  Value=500
  BW Cycles Since Last CEB : Integrator  ExternalReset=rising  InitialConditionSource=external  InitialCondition=5
  BW Maintenance Request Signal : RelationalOperator  OutDataTypeStr=boolean  RndMeth=Simplest  InputSameDT=off
  BW Maintenance Setpoint (min) : Constant  Value=55
  Bus Selector : BusSelector  OutputSignals=UF_FeedTemperature_degC,UF_FeedTurbidity_NTU
  Bus Selector1 : BusSelector  OutputSignals=UF9_MaintenanceCompletion_signal,UF9_OperationsState_signal
  Bus Selector3 : BusSelector  OutputSignals=UF9_FeedFlow,UF_FeedPressure_psi
  CEBSignal_Level : Gain  Gain=2  OutDataTypeStr=double
  Compare To Constant : simulink/Logic and Bit Operations/Compare To Constant  relop=>  const=10  OutDataTypeStr=boolean
  Data Type Conversion : DataTypeConversion  SaturateOnIntegerOverflow=off  RndMeth=Floor
  Data Type Conversion1 : DataTypeConversion  SaturateOnIntegerOverflow=off  RndMeth=Floor
  Filtrate Flow Rate : Product
  Filtrate Pressure MAX (psi) : Constant  Value=39
  Filtrate Pressure Ratio (dmnl) : Constant  Value=.89
  GreaterThanOrEqual : RelationalOperator  OutDataTypeStr=boolean  RndMeth=Simplest  InputSameDT=off
  Memory : Memory
  MergeSignals : Sum  Inputs=|++
  Minus : Sum  Inputs=+-
  NOT : Logic  Operator=NOT  IconShape=distinctive  AllPortsSameDT=off  OutDataTypeStr=boolean
  Product : Product
  Product1 : Product
  Ramping Permeate Pressure : MinMax  Inputs=2
  Scope : Scope  NumInputPorts=3
      settings: ActiveDisplayYMinimum=-126.71796384165732  ActiveDisplayYMaximum=1140.4616745749161  DataLoggingVariableName=ScopeData10
  Scope1 : Scope  NumInputPorts=2
      settings: ActiveDisplayYMinimum=-129.2228584451866  ActiveDisplayYMaximum=1163.0057260066797  DataLoggingVariableName=ScopeData11
  Step Add (min) : Constant
  Subsystem : Subsystem
  TEST : Scope  NumInputPorts=4
      settings: ActiveDisplayYMinimum=13.625  ActiveDisplayYMaximum=27.375  DataLoggingVariableName=ScopeData3
  TEST2 : Scope  NumInputPorts=2
      settings: ActiveDisplayYMinimum=-311929.86683332996  ActiveDisplayYMaximum=2.8073688014999703E+6  DataLoggingVariableName=ScopeData4
  TMP (psi) : Sum  Inputs=|-+
  Time Since Last Backwash (min) : Integrator  ExternalReset=level hold  InitialConditionSource=external  InitialCondition=26
  Time Since Last CEB (min) : Integrator  ExternalReset=level hold  InitialConditionSource=external  InitialCondition=4833
  Time Since Last CIP (min) : Integrator  InitialCondition=round(CIP_Max_Time*rand())
  Time in Operation (only while running) : Product
  UF9_BWCompleteSignal : simulink/Logic and Bit Operations/Compare To Constant  relop===  const=1  OutDataTypeStr=uint8
  UF9_BWCycles_InitCondition : Step  Before=round(500 * rand())  After=0  SampleTime=0
  UF9_BWQualification : Logic  IconShape=distinctive  AllPortsSameDT=off  OutDataTypeStr=boolean
  UF9_BWTime_InitCondition : Step  Before=round(BW_Max_Time*rand())  After=0  SampleTime=0
  UF9_BWVol_InitCondition : Step  Before=round(BW_Max_Vol_gal*rand())  After=0  SampleTime=0
  UF9_CEBCompleteSignal : simulink/Logic and Bit Operations/Compare To Constant  relop===  const=2  OutDataTypeStr=uint8
  UF9_CEBQualification : Logic  IconShape=distinctive  AllPortsSameDT=off  OutDataTypeStr=boolean
  UF9_CEBTime_InitCondition : Step  Before=round(CEB_Max_Time*rand())  After=0  SampleTime=0
  UF9_CEBVol_InitCondition : Step  Before=round(CEB_Max_Vol_gal*rand())  After=0  SampleTime=0
  Volume Since Last Backwash (gal) : Integrator  ExternalReset=level hold  InitialConditionSource=external  InitialCondition=34330
  Volume Since Last CEB (gal) : Integrator  ExternalReset=rising  InitialConditionSource=external  InitialCondition=2777254
  "gpd -> gpm/psi" : Gain  Gain=1/1440
  Filtrate Flow (gpm) : Outport
  tag scope: UF9_Maintenance_Request=global, UF9_PermeatePressure_psi=global, UF9_gpm_psi=global
  wires:
  Volume Since Last Backwash (gal)/1 -> Subsystem/4(V_BW), TEST2/1  "V_BW"
  Time Since Last Backwash (min)/1 -> BW Maintenance Request Signal/1, Subsystem/1(t_BW), TEST/1
  Product/1 -> "gpd -> gpm/psi"/1  "UF Spec. Flow (gpd/psi)"
  [UF_MembraneCharacteristics] -> Product/2  "Membrane Area (ft^2)"
  "gpd -> gpm/psi"/1 -> Filtrate Flow Rate/1, [UF9_gpm_psi]  "Water Permeability (gpm/psi)"
  Time in Operation (only while running)/1 -> Time Since Last Backwash (min)/1, Time Since Last CEB (min)/1, Time Since Last CIP (min)/1
  Filtrate Flow Rate/1 -> Scope/1, Minus/2, Volume Since Last Backwash (gal)/1, Volume Since Last CEB (gal)/1, Compare To Constant/1, Filtrate Flow (gpm)/1  "UF9 Filtrate Flow (gpm)"
  Time Since Last CEB (min)/1 -> Subsystem/2(t_CEB), TEST/2  "t_CEB"
  Volume Since Last CEB (gal)/1 -> Subsystem/5(V_CEB), TEST2/2  "V_CEB"
  Time Since Last CIP (min)/1 -> Subsystem/3(t_CIP), TEST/3  "t_CIP"
  Filtrate Pressure MAX (psi)/1 -> Ramping Permeate Pressure/1
  [UF_Influent_WQ] -> Bus Selector/1
  Bus Selector/1 -> Subsystem/7(T)  "<UF_FeedTemperature_degC>"
  UF9_FeedFlow_Pressure/1 -> Bus Selector3/1
  Filtrate Pressure Ratio (dmnl)/1 -> Product1/1
  Product1/1 -> Ramping Permeate Pressure/2
  Ramping Permeate Pressure/1 -> [UF9_PermeatePressure_psi], TMP (psi)/1
  TMP (psi)/1 -> Filtrate Flow Rate/2
  BW Maintenance Setpoint (min)/1 -> BW Maintenance Request Signal/2
  BW Cycles Since Last CEB/1 -> GreaterThanOrEqual/1
  BW Cycles Setpoint/1 -> GreaterThanOrEqual/2
  Bus Selector/2 -> Subsystem/6(Feed Turbidity)  "<UF_FeedTurbidity_NTU>"
  [UF9_State] -> Bus Selector1/1
  MergeSignals/1 -> [UF9_Maintenance_Request]  "UF9_MaintenanceRequest"
  UF9_CEBCompleteSignal/1 -> Data Type Conversion1/1  "CEBCompleteSignal"
  [CEBCompleteSignal] -> Volume Since Last CEB (gal)/2, Time Since Last CEB (min)/2
  Data Type Conversion/1 -> [BWCompleteSignal], BW Cycles Since Last CEB/1  "BWCompleteSignal"
  [BWCompleteSignal] -> Volume Since Last Backwash (gal)/2, Time Since Last Backwash (min)/2
  [CEBCompleteSignal] -> BW Cycles Since Last CEB/2
  Bus Selector1/1 -> Memory/1  "<UF9_MaintenanceCompletion_signal>"
  UF9_BWCompleteSignal/1 -> Data Type Conversion/1  "BWCompleteSignal"
  Data Type Conversion1/1 -> [CEBCompleteSignal]  "CEBCompleteSignal"
  UF9_BWCycles_InitCondition/1 -> BW Cycles Since Last CEB/3
  Subsystem/1(A_UF) -> TEST/4, Product/1  "membrane permeability (GFD/psi)"
  UF9_BWTime_InitCondition/1 -> Time Since Last Backwash (min)/3  "T_BWInitCondition"
  UF9_CEBVol_InitCondition/1 -> Volume Since Last CEB (gal)/3
  UF9_CEBTime_InitCondition/1 -> Time Since Last CEB (min)/3
  UF9_BWVol_InitCondition/1 -> Volume Since Last Backwash (gal)/3  "V_BWInitCondition"
  Step Add (min)/1 -> Time in Operation (only while running)/1
  Compare To Constant/1 -> Time in Operation (only while running)/2
  Memory/1 -> UF9_BWCompleteSignal/1, UF9_CEBCompleteSignal/1
  UF9_BWQualification/1 -> MergeSignals/1  "UF9_BWRequest"
  GreaterThanOrEqual/1 -> UF9_CEBQualification/2  "UF9 CEB Request Signal"
  UF9_CEBQualification/1 -> CEBSignal_Level/1, NOT/1  "UF9_CEBRequest"
  BW Maintenance Request Signal/1 -> UF9_BWQualification/1, UF9_CEBQualification/1  "UF9 BW Request Signal"
  NOT/1 -> UF9_BWQualification/2
  CEBSignal_Level/1 -> MergeSignals/2  "UF9_CEBRequest"
  Bus Selector3/1 -> Scope1/2, Minus/1, Scope/3  "<UF9_FeedFlow>"
  Bus Selector3/2 -> TMP (psi)/2, Scope1/1, Product1/2  "<UF_FeedPressure_psi>"
  Minus/1 -> Scope/2  "WasteFlow_UF9"

== system Ultrafiltration/UF_Feed_Manifold ==
  Bus Creator{,1..10} (11 alike) : BusCreator  Inputs=2
  Constant3 : Constant  Value=400
  Demux : Demux  Outputs=10
  Demux1 : Demux  Outputs=10
  Display1 : Display
  Feed Turbidity (NTU) : Constant  Value=.4194
  MATLAB Function : MATLAB Function  TreatAsAtomicUnit=on
  Mux : Mux  Inputs=10
  Mux1 : Mux  Inputs=10
  Mux2 : Mux  Inputs=10
  Scope : Scope  NumInputPorts=3
      settings: ActiveDisplayYMinimum=-2.1636362137691987  ActiveDisplayYMaximum=19.472725923922791  DataLoggingVariableName=ScopeData5
  Scope1 : Scope
      settings: ActiveDisplayYMinimum=-1.4451216634885196  ActiveDisplayYMaximum=13.006094971396678  DataLoggingVariableName=ScopeData6
  Scope2 : Scope
      settings: DataLoggingVariableName=ScopeData9
  Temperature (oC) : Constant  Value=22.4133
  To UF1 : Outport
  To UF2 : Outport  Port=2
  To UF3 : Outport  Port=3
  To UF4 : Outport  Port=4
  To UF5 : Outport  Port=5
  To UF6 : Outport  Port=6
  To UF7 : Outport  Port=7
  To UF8 : Outport  Port=8
  To UF9 : Outport  Port=9
  To UF10 : Outport  Port=10
  tag scope: UF_Influent_WQ=global
  wires:
  Bus Creator5/1 -> To UF5/1
  Bus Creator2/1 -> To UF2/1
  Temperature (oC)/1 -> Bus Creator/1  "UF_FeedTemperature_degC"
  Demux/6 -> Bus Creator6/1  "UF6_FeedFlow"
  Feed Turbidity (NTU)/1 -> Bus Creator/2  "UF_FeedTurbidity_NTU"
  [UF1_gpm_psi] -> Mux/1
  Demux/3 -> Bus Creator3/1  "UF3_FeedFlow"
  Constant3/1 -> Mux/3, Mux/2, Mux/4, Mux/5, Mux/6, Mux/7, Mux/8, Mux/9, Mux/10
  [UF4_gpm_psi] -> Mux1/4
  [UF2_gpm_psi] -> Mux1/2
  [UF1_gpm_psi] -> Mux1/1
  [UF10_PermeatePressure_psi] -> Mux2/10
  [UF3_gpm_psi] -> Mux1/3
  [UF4_PermeatePressure_psi] -> Mux2/4
  [UF5_gpm_psi] -> Mux1/5
  [UF6_gpm_psi] -> Mux1/6
  [UF3_PermeatePressure_psi] -> Mux2/3
  [UF7_gpm_psi] -> Mux1/7
  [UF5_PermeatePressure_psi] -> Mux2/5
  [UF8_gpm_psi] -> Mux1/8
  [UF9_gpm_psi] -> Mux1/9
  [UF10_gpm_psi] -> Mux1/10
  Bus Creator3/1 -> To UF3/1
  [UF1_PermeatePressure_psi] -> Mux2/1
  Demux1/3 -> Bus Creator3/2  "UF_FeedPressure_psi"
  MATLAB Function/3(dP_valve_req) -> Scope1/1
  [UF2_PermeatePressure_psi] -> Mux2/2
  Bus Creator4/1 -> To UF4/1
  Demux1/5 -> Bus Creator5/2  "UF_FeedPressure_psi"
  [UF6_PermeatePressure_psi] -> Mux2/6
  [UF7_PermeatePressure_psi] -> Mux2/7
  [UF_Flow_Assignment] -> Scope/2, Demux/1, MATLAB Function/1(prescribed_feedflow_vec)
  [UF8_PermeatePressure_psi] -> Mux2/8
  [UF9_PermeatePressure_psi] -> Mux2/9
  Bus Creator/1 -> [UF_Influent_WQ]
  Demux1/4 -> Bus Creator4/2  "UF_FeedPressure_psi"
  Demux/4 -> Bus Creator4/1  "UF4_FeedFlow"
  Mux1/1 -> MATLAB Function/2(membrane_conductance_vec)
  Mux2/1 -> MATLAB Function/3(UF_PermeatePressure_vec)  "psi"
  MATLAB Function/1(UF_FeedPressure_vector) -> Demux1/1, Scope/1
  MATLAB Function/2(UFPump_Pressure_Setpoint) -> Display1/1, Scope/3
  Demux/1 -> Bus Creator1/1  "UF1_FeedFlow"
  Bus Creator1/1 -> To UF1/1
  Demux/2 -> Bus Creator2/1  "UF2_FeedFlow"
  Demux/5 -> Bus Creator5/1  "UF5_FeedFlow"
  Demux1/1 -> Bus Creator1/2  "UF_FeedPressure_psi"
  Demux1/2 -> Bus Creator2/2  "UF_FeedPressure_psi"
  Demux1/6 -> Bus Creator6/2  "UF_FeedPressure_psi"
  Bus Creator6/1 -> To UF6/1
  Bus Creator7/1 -> To UF7/1
  Demux1/7 -> Bus Creator7/2  "UF_FeedPressure_psi"
  Demux/7 -> Bus Creator7/1  "UF7_FeedFlow"
  Bus Creator8/1 -> To UF8/1
  Demux1/8 -> Bus Creator8/2  "UF_FeedPressure_psi"
  Demux/8 -> Bus Creator8/1  "UF8_FeedFlow"
  Bus Creator9/1 -> To UF9/1
  Demux1/9 -> Bus Creator9/2  "UF_FeedPressure_psi"
  Demux/9 -> Bus Creator9/1  "UF9_FeedFlow"
  Bus Creator10/1 -> To UF10/1
  Demux1/10 -> Bus Creator10/2  "UF_FeedPressure_psi"
  Demux/10 -> Bus Creator10/1  "UF10_FeedFlow"
